simulink model "RealWorld"  (R2024b)
settings: Solver=VariableStepAuto  StartTime=0.0  StopTime=10.0  RelTol=1e-3
undefined symbols (not defined in the file or in its folder): env, flag, IC, orb, sat, sens
libraries: matrix_library x8, vrlib x1
(part 1 of 2)
settings Model: Creator=filippocamaleonte  LastModifiedBy=eleon

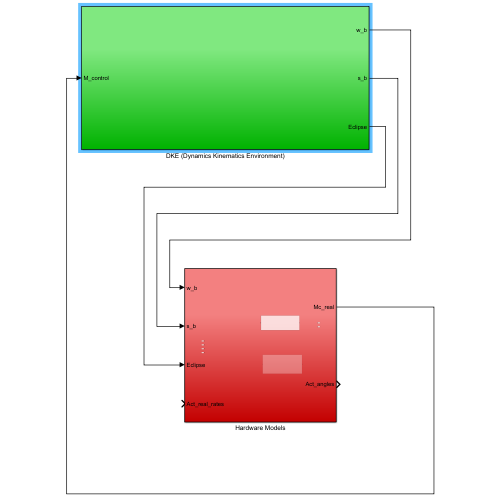
[thumbnail: Simulink's stored preview of the top-level diagram]
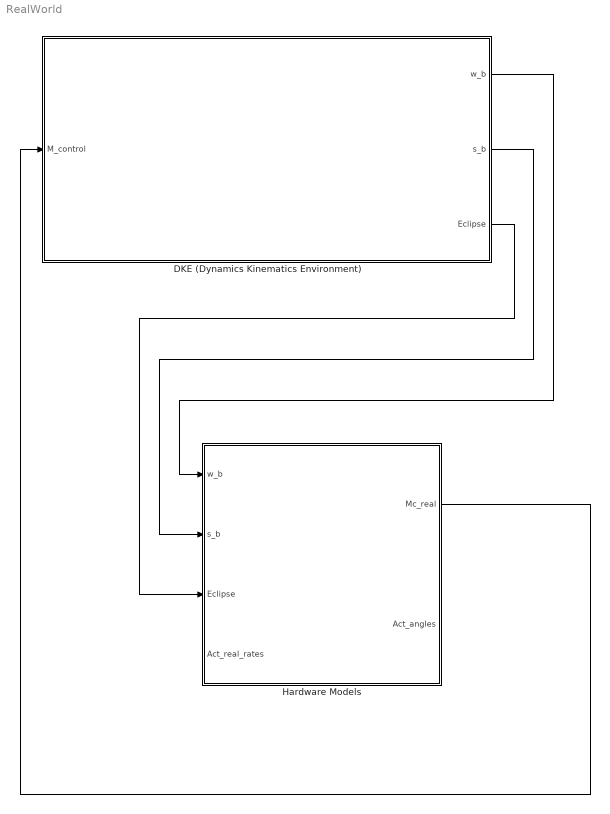
== system RealWorld ==
  DKE (Dynamics Kinematics Environment) : Subsystem
  Hardware Models : Subsystem
  wires:
  DKE (Dynamics Kinematics Environment)/2(s_b) -> Hardware Models/2(s_b)
  DKE (Dynamics Kinematics Environment)/3(Eclipse) -> Hardware Models/3(Eclipse)
  DKE (Dynamics Kinematics Environment)/1(w_b) -> Hardware Models/1(w_b)
  Hardware Models/1(Mc_real) -> DKE (Dynamics Kinematics Environment)/1(M_control)

== system RealWorld/DKE (Dynamics Kinematics Environment) ==
  M_control : Inport
  Dynamics : Subsystem
  Environment : Subsystem
  Kinematics : Subsystem
  Sum : Sum  Inputs=|++
  w_b : Outport
  s_b : Outport  Port=2
  Eclipse : Outport  Port=3
  wires:
  M_control/1 -> Sum/1
  Dynamics/1(w_b) -> [w_b], Kinematics/1(w_b)
  Sum/1 -> Dynamics/1(M_ext)
  Environment/3(Disturbance_torque) -> Sum/2
  [w_b] -> w_b/1
  Environment/1(Eclipse) -> Eclipse/1
  Kinematics/3(r_n) -> Environment/3(r_n)
  Kinematics/1(A_bn) -> Environment/1(A_bn)
  Kinematics/2(A_bl) -> Environment/2(A_bl)

== system RealWorld/Hardware Models ==
  w_b : Inport
  s_b : Inport  Port=2
  Eclipse : Inport  Port=3
  Act_real_rates : Inport  Port=4
  Actuators : Subsystem
  Sensors : Subsystem  Commented=on
  Mc_real : Outport
  Act_angles : Outport  Port=2

== system RealWorld/DKE (Dynamics Kinematics Environment)/Dynamics ==
  note: Here we need both Newton and Euler Law
  M_ext : Inport
  Euler Integrator : Subsystem
  w_b : Outport
  wires:
  M_ext/1 -> Euler Integrator/1(M_ext)
  Euler Integrator/1(w_b) -> w_b/1

== system RealWorld/DKE (Dynamics Kinematics Environment)/Environment ==
  note: Enviroment Models (Celestial Objects, Shadow, Magnetic Field, atmosphere, albedo)
  A_bn : Inport
  A_bl : Inport  Port=2
  r_n : Inport  Port=3
  Conical Shadow Model : Subsystem
  MatrixMultiply : Product  Multiplication=Matrix(*)
  Perturbations : Subsystem
  Sun Direction Circular Orbit : Subsystem
  Eclipse : Outport
  s_n : Outport  Port=2
  Disturbance_torque : Outport  Port=3
  wires:
  Sun Direction Circular Orbit/1(S_n) -> [S_n], s_n/1, Conical Shadow Model/1(S_n)
  Conical Shadow Model/1(eclipseFlag) -> Eclipse/1
  Perturbations/1(Disturbance_torque) -> Disturbance_torque/1
  r_n/1 -> Perturbations/2(r_n), Conical Shadow Model/2(r_n)
  A_bn/1 -> MatrixMultiply/1
  [S_n] -> MatrixMultiply/2
  MatrixMultiply/1 -> Perturbations/1(S_b)  "S_b"
  A_bl/1 -> Perturbations/3(A_bl)

== system RealWorld/DKE (Dynamics Kinematics Environment)/Kinematics ==
  note: B/N calculation
      | Keplerian calculations
      | L/N calculation
      | B/L calculation
  w_b : Inport
  Attitude Error : Subsystem
  Constant1 : Constant  Value=orb.i
  EulerKinematicsdelay : Subsystem
  Kepler Integrator1 : Subsystem
  LVLH Evolution wtr of Earth : Subsystem
  SpaceCraft position wrt ECI : Subsystem
  A_bn : Outport
  A_bl : Outport  Port=2
  r_n : Outport  Port=3
  wires:
  w_b/1 -> EulerKinematicsdelay/1(w_b)
  Attitude Error/1(A_bl) -> A_bl/1
  EulerKinematicsdelay/1(A_bn) -> A_bn/1, Attitude Error/1(A_bn)
  LVLH Evolution wtr of Earth/1(A_ln) -> Attitude Error/2(A_ln)
  Constant1/1 -> LVLH Evolution wtr of Earth/2(i)
  Kepler Integrator1/1(th) -> SpaceCraft position wrt ECI/1(th), LVLH Evolution wtr of Earth/1(th)
  SpaceCraft position wrt ECI/1(r_n) -> r_n/1

== system RealWorld/Hardware Models/Actuators ==
  In1 : Inport
  Out1 : Outport
  wires:
  In1/1 -> Out1/1

== system RealWorld/Hardware Models/Sensors ==
  note: Sun Sensors Array
  In1 : Inport
  Gyroscope : Subsystem
  Sun Sensor (S1) : Subsystem
  Sun Sensor (S2) : Subsystem
  Sun Sensor (S3) : Subsystem
  Sun Sensor (S4) : Subsystem
  Out1 : Outport

== system RealWorld/DKE (Dynamics Kinematics Environment)/Dynamics/Euler Integrator ==
  M_ext : Inport
  Constant : Constant  Value=sat.I
  Constant1 : Constant  Value=sat.w0  VectorParams1D=off
  Constant2 : Constant  Value=sat.invI
  Cross Product : matrix_library/Cross Product
  Divide : Product  Inputs=**  Multiplication=Matrix(*)
  Integrator : Integrator  InitialConditionSource=external
  Product : Product  Multiplication=Matrix(*)
  Sum : Sum  Inputs=|++
  w_b : Outport
  wires:
  Product/1 -> Cross Product/1
  Divide/1 -> Integrator/1
  Constant/1 -> Product/1
  Constant2/1 -> Divide/1
  Integrator/1 -> Product/2, Cross Product/2, w_b/1
  Constant1/1 -> Integrator/2
  Cross Product/1 -> Sum/1
  Sum/1 -> Divide/2
  M_ext/1 -> Sum/2

== system RealWorld/DKE (Dynamics Kinematics Environment)/Environment/Conical Shadow Model ==
  note: Output Interface
  note: Input Interface
  note: Model is cylindrical shadow, formula was taken by Crassidis
  S_n : Inport
  r_n : Inport  Port=2
  Dot Product : DotProduct  OutDataTypeStr=Inherit: Inherit via internal rule
  Earth's Radius : Constant  Value=env.Earth.R
  Eclipse (1) : Subsystem  TreatAsAtomicUnit=on
  Gain : Gain  Gain=-1
  If : If  NumInputs=2  IfExpression=u1 < u2
  Merge : Merge
  Norm : Subsystem
  NotEclipse (0) : Subsystem  TreatAsAtomicUnit=on
  Sqrt : Sqrt
  Square : Math  Operator=square
  Square1 : Math  Operator=square
  Subtract : Sum  Inputs=+-
  eclipseFlag : Outport
  wires:
  r_n/1 -> Dot Product/2, Norm/1(Vector)  "r_n"
  S_n/1 -> Dot Product/1  "S_n"
  Norm/1(Norm) -> Square1/1  "norm_r"
  If/1 -> Eclipse (1)/Action
  If/2 -> NotEclipse (0)/Action
  Merge/1 -> eclipseFlag/1
  Eclipse (1)/1(One) -> Merge/1
  NotEclipse (0)/1(Zero) -> Merge/2
  Dot Product/1 -> If/1
  Gain/1 -> If/2
  Sqrt/1 -> Gain/1
  Subtract/1 -> Sqrt/1
  Square/1 -> Subtract/2
  Square1/1 -> Subtract/1
  Earth's Radius/1 -> Square/1  "earth_R"

== system RealWorld/DKE (Dynamics Kinematics Environment)/Environment/Perturbations ==
  note: Gravity Gradiente
      | Solar Pressure
      | Magnetic torquer
      | Air drag ??
  S_b : Inport
  r_n : Inport  Port=2
  A_bl : Inport  Port=3
  Gravity Gradient Torque : Subsystem
  Magnetic Field order 1 : Subsystem
  Solar Radiation Pressure Torque : Subsystem
  Sum : Sum  Inputs=++++
  Disturbance_torque : Outport
  wires:
  Sum/1 -> Disturbance_torque/1
  Solar Radiation Pressure Torque/1(T_srp) -> Sum/2
  S_b/1 -> Solar Radiation Pressure Torque/1(S_b)
  A_bl/1 -> Gravity Gradient Torque/1(A_bl)
  r_n/1 -> Gravity Gradient Torque/2(r_n)
  Gravity Gradient Torque/1(T_gg) -> Sum/1

== system RealWorld/DKE (Dynamics Kinematics Environment)/Environment/Sun Direction Circular Orbit ==
  note: Input Interface
  note: Output Interface
  Clock : Clock
  Cos : Trigonometry  Operator=cos
  Cos1 : Trigonometry  Operator=cos
  Earth's Inclination : Constant  Value=env.Earth.i
  Gain : Gain  Gain=env.Earth.n
  Matrix Concatenate : Concatenate  NumInputs=3  Mode=Multidimensional array
  Product : Product
  Product1 : Product
  Product2 : Product
  Sin : Trigonometry
  Sin1 : Trigonometry
  Sun's Radius : Constant  Value=env.Sun.R
  S_n : Outport
  wires:
  Clock/1 -> Gain/1
  Gain/1 -> Sin/1, Cos/1
  Product/1 -> S_n/1
  Sun's Radius/1 -> Product/2
  Matrix Concatenate/1 -> Product/1
  Earth's Inclination/1 -> Sin1/1, Cos1/1
  Cos1/1 -> [cos]
  Sin1/1 -> [sin]
  Cos/1 -> Matrix Concatenate/1
  Product1/1 -> Matrix Concatenate/2
  Product2/1 -> Matrix Concatenate/3
  [sin] -> Product2/2
  [cos] -> Product1/1
  Sin/1 -> Product1/2, Product2/1

== system RealWorld/DKE (Dynamics Kinematics Environment)/Kinematics/Attitude Error ==
  A_bn : Inport
  A_ln : Inport  Port=2
  Matrix Multiply : Product  Multiplication=Matrix(*)
  Transpose : Math  Operator=transpose
  A_bl : Outport
  wires:
  Transpose/1 -> Matrix Multiply/2
  A_ln/1 -> Transpose/1
  Matrix Multiply/1 -> A_bl/1
  A_bn/1 -> Matrix Multiply/1

== system RealWorld/DKE (Dynamics Kinematics Environment)/Kinematics/EulerKinematicsdelay ==
  note: Logic
  note: The flag is set to -1 when 313 is used and to 1 when 312 is used
  w_b : Inport
  312 Propagator : Subsystem
  312To313 : Subsystem
  313 Propagator : Subsystem
  313To312 : Subsystem
  A312 : Subsystem
  A313 : Subsystem
  Abs : Abs  SaturateOnIntegerOverflow=off
  Cos : Trigonometry  Operator=cos
  IC : InitialCondition  Value=IC.angles
  IC1 : InitialCondition  Value=IC.angles
  IC3 : InitialCondition
  Relay : Relay  OnSwitchValue=0.75  OffSwitchValue=0.35  OffOutputValue=-1
  Selector1 : Selector  InputPortWidth=3  IndexOptions=Index vector (dialog)  Indices=[2]  OutputSizes=1
  Switch : Switch  Criteria=u2 > Threshold  SaturateOnIntegerOverflow=off  InputSameDT=off
  Switch1 : Switch  Criteria=u2 > Threshold  SaturateOnIntegerOverflow=off  InputSameDT=off
  To Workspace : ToWorkspace  VariableName=flag1  SampleTime=-1
  To Workspace1 : ToWorkspace  VariableName=eu312  SampleTime=-1
  To Workspace2 : ToWorkspace  VariableName=eu313  SampleTime=-1
  A_bn : Outport
  wires:
  Cos/1 -> Abs/1
  Selector1/1 -> Cos/1
  Abs/1 -> Relay/1
  A313/1(Out1) -> Switch/3
  w_b/1 -> 313 Propagator/2(w_b), 312 Propagator/2(w_b)  "w_b"
  313 Propagator/1(EA) -> [Euler313], A313/1(Euler Angles)  "EulerAngles313"
  A312/1(DCM) -> Switch/1
  Switch1/1 -> Selector1/1
  Switch/1 -> A_bn/1  "DCM"
  313To312/1(Out1) -> IC1/1
  312To313/1(Out1) -> IC/1
  IC1/1 -> 312 Propagator/1(IC)
  IC/1 -> 313 Propagator/3(IC)
  [EulerFlag] -> Switch/2, 312 Propagator/3(Reset), 313 Propagator/1(Reset)
  312 Propagator/1(EA) -> [Euler312], A312/1(Euler Angles)  "EulerAngles312"
  312 Propagator/2(Out1) -> 312To313/1(In1)
  313 Propagator/2(Out1) -> 313To312/1(In1)
  Relay/1 -> IC3/1
  [Euler312] -> To Workspace1/1, Switch1/1
  [Euler313] -> To Workspace2/1, Switch1/3
  [EulerFlag] -> Switch1/2
  IC3/1 -> To Workspace/1, [EulerFlag]

== system RealWorld/DKE (Dynamics Kinematics Environment)/Kinematics/Kepler Integrator1 ==
  Add : Sum  Inputs=+-
  Add1 : Sum
  Constant : Constant  Value=IC.theta
  Constant1 : Constant  Value=3/2
  Constant2 : Constant
  Constant3 : Constant  Value=2
  Constant4 : Constant  Value=orb.e
  Constant5 : Constant  Value=2
  Constant6 : Constant
  Cosh : Trigonometry  Operator=cos
  Divide : Product  Inputs=*/
  Gain : Gain  Gain=orb.n
  Gain1 : Gain  Gain=orb.e
  Integrator : Integrator  InitialConditionSource=external  WrapState=on  WrappedStateUpperValue=2*pi  WrappedStateLowerValue=0
  Power : Math  Operator=pow
  Power1 : Math  Operator=pow
  Power2 : Math  Operator=pow
  th : Outport
  wires:
  Constant/1 -> Integrator/2
  Integrator/1 -> Cosh/1, th/1
  Divide/1 -> Integrator/1
  Power/1 -> Divide/2
  Constant1/1 -> Power/2
  Constant2/1 -> Add/1
  Add/1 -> Power/1
  Power1/1 -> Add/2
  Constant3/1 -> Power1/2
  Constant4/1 -> Power1/1
  Gain/1 -> Divide/1
  Power2/1 -> Gain/1
  Constant5/1 -> Power2/2
  Add1/1 -> Power2/1
  Constant6/1 -> Add1/1
  Gain1/1 -> Add1/2
  Cosh/1 -> Gain1/1

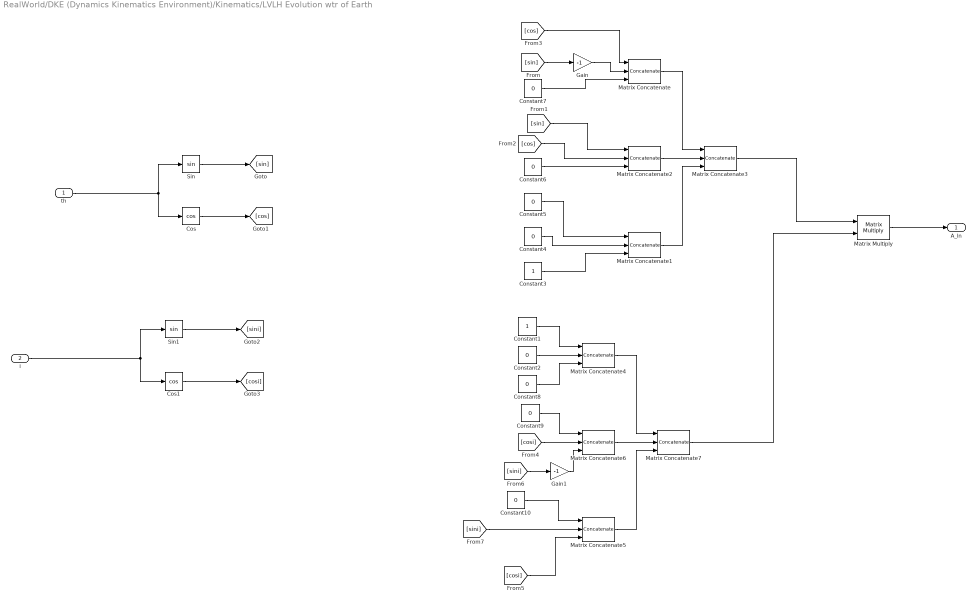
== system RealWorld/DKE (Dynamics Kinematics Environment)/Kinematics/LVLH Evolution wtr of Earth ==
  th : Inport
  i : Inport  Port=2
  Constant1 : Constant
  Constant{2,4..10} (8 alike) : Constant  Value=0
  Constant3 : Constant
  Cos : Trigonometry  Operator=cos
  Cos1 : Trigonometry  Operator=cos
  Gain : Gain  Gain=-1
  Gain1 : Gain  Gain=-1
  Matrix Concatenate{,1..2,4..6} (6 alike) : Concatenate  NumInputs=3  Mode=Multidimensional array
  Matrix Concatenate3 : Concatenate  NumInputs=3  Mode=Multidimensional array  ConcatenateDimension=2
  Matrix Concatenate7 : Concatenate  NumInputs=3  Mode=Multidimensional array  ConcatenateDimension=2
  Matrix Multiply : Product  Multiplication=Matrix(*)
  Sin : Trigonometry
  Sin1 : Trigonometry
  A_ln : Outport
  wires:
  Cos/1 -> [cos]
  Matrix Concatenate1/1 -> Matrix Concatenate3/3
  th/1 -> Cos/1, Sin/1
  Matrix Concatenate/1 -> Matrix Concatenate3/1
  Constant5/1 -> Matrix Concatenate1/1
  Constant3/1 -> Matrix Concatenate1/3
  [cos] -> Matrix Concatenate/1
  Sin/1 -> [sin]
  Constant6/1 -> Matrix Concatenate2/3
  Constant7/1 -> Matrix Concatenate/3
  Constant4/1 -> Matrix Concatenate1/2
  Matrix Concatenate2/1 -> Matrix Concatenate3/2
  [cos] -> Matrix Concatenate2/2
  [sin] -> Matrix Concatenate2/1
  Gain/1 -> Matrix Concatenate/2
  [sin] -> Gain/1
  Cos1/1 -> [cosi]
  Sin1/1 -> [sini]
  i/1 -> Cos1/1, Sin1/1
  Matrix Multiply/1 -> A_ln/1
  Matrix Concatenate3/1 -> Matrix Multiply/1
  Matrix Concatenate7/1 -> Matrix Multiply/2
  Matrix Concatenate6/1 -> Matrix Concatenate7/2
  Matrix Concatenate5/1 -> Matrix Concatenate7/3
  Matrix Concatenate4/1 -> Matrix Concatenate7/1
  Constant1/1 -> Matrix Concatenate4/1
  Constant2/1 -> Matrix Concatenate4/2
  Constant8/1 -> Matrix Concatenate4/3
  Constant9/1 -> Matrix Concatenate6/1
  Constant10/1 -> Matrix Concatenate5/1
  [cosi] -> Matrix Concatenate5/3
  [cosi] -> Matrix Concatenate6/2
  [sini] -> Matrix Concatenate5/2
  [sini] -> Gain1/1
  Gain1/1 -> Matrix Concatenate6/3

== system RealWorld/DKE (Dynamics Kinematics Environment)/Kinematics/SpaceCraft position wrt ECI ==
  th : Inport
  Add : Sum
  Add1 : Sum  Inputs=+-
  Constant : Constant  Value=orb.i
  Constant1 : Constant  Value=orb.i
  Constant2 : Constant
  Constant3 : Constant
  Constant4 : Constant  Value=2
  Constant5 : Constant  Value=orb.e
  Cos : Trigonometry  Operator=cos
  Cos1 : Trigonometry  Operator=cos
  Cos2 : Trigonometry  Operator=cos
  Divide : Product  Inputs=*/
  Gain : Gain  Gain=orb.e
  Gain1 : Gain  Gain=orb.a
  Matrix Concatenate : Concatenate  NumInputs=3  Mode=Multidimensional array
  Power : Math  Operator=pow
  Product : Product
  Product1 : Product
  Product2 : Product
  Sin : Trigonometry
  Sin1 : Trigonometry
  r_n : Outport
  wires:
  Constant/1 -> Sin/1
  Cos1/1 -> Matrix Concatenate/1
  th/1 -> Sin1/1, Cos2/1, Cos1/1
  Product1/1 -> Matrix Concatenate/2
  Product/1 -> Matrix Concatenate/3
  Sin1/1 -> Product1/2, Product/1
  Sin/1 -> Product/2
  Constant1/1 -> Cos/1
  Cos/1 -> Product1/1
  Product2/1 -> r_n/1
  Matrix Concatenate/1 -> Product2/1
  Divide/1 -> Product2/2
  Constant2/1 -> Add/1
  Add/1 -> Divide/2
  Cos2/1 -> Gain/1
  Gain/1 -> Add/2
  Constant3/1 -> Add1/1
  Power/1 -> Add1/2
  Constant4/1 -> Power/2
  Constant5/1 -> Power/1
  Add1/1 -> Gain1/1
  Gain1/1 -> Divide/1

== system RealWorld/Hardware Models/Sensors/Gyroscope ==
  note: Sensor Model
  note: Noise Model
  note: Input Interface
  note: G sensing Model
  note: Sources:
      | - Crassidis
      | - Giacomo Langfelder Course
      | - Colagrossi's book
      | - Safran STIM210 Datasheet
      |
      | To Do:
      | Add Temperature model and more precise dealy model
  note: We assume that the Sensor is Oriented in the same axis as the body
  note: Output Interface
  w_b : Inport
  a_b : Inport  Port=2
  Add : Sum  Inputs=++++
  Add1 : Sum
  Constant : Constant  Value=flag.realsensors
  Constant1 : Constant  Value=sens.gyro.scaleFactor
  Constant2 : Constant  Value=sens.gyro.orth
  Constant3 : Constant  Value=sens.gyro.missalign
  Constant4 : Constant  Value=sens.gyro.bias
  Constant5 : Constant  Value=sens.gyro.gsensing
  Discrete Transfer Fcn : DiscreteTransferFcn  Numerator=1  Denominator=[1 0.8]
  MatrixMultiply{,1..3} (4 alike) : Product  Multiplication=Matrix(*)
  Quantizer : Quantizer  QuantizationInterval=sens.gyro.ADC.quanta
  Random Number : RandomNumber  Variance=sens.gyro.biasInstability  SampleTime=1/sens.gyro.freq
  Random Number1 : RandomNumber  Variance=sens.gyro.arw  SampleTime=1/sens.gyro.freq
  Saturation : Saturate  UpperLimit=sens.gyro.saturation  LowerLimit=-sens.gyro.saturation
  Scope : Scope  NumInputPorts=2
  Scope1 : Scope
  Scope2 : Scope  NumInputPorts=2
  Switch : Switch  Criteria=u2 > Threshold  SaturateOnIntegerOverflow=off  InputSameDT=off
  Zero-Order Hold : ZeroOrderHold  SampleTime=1/sens.gyro.freq
  w_meas_b : Outport
  wires:
  Switch/1 -> w_meas_b/1
  Constant/1 -> Switch/2
  [w_meas_b] -> Switch/1
  [w_b] -> Switch/3
  w_b/1 -> [w_b]
  Quantizer/1 -> [w_meas_b]
  Zero-Order Hold/1 -> Quantizer/1
  Saturation/1 -> Zero-Order Hold/1
  MatrixMultiply/1 -> MatrixMultiply1/1
  MatrixMultiply1/1 -> MatrixMultiply2/1
  Constant1/1 -> MatrixMultiply/1
  Constant2/1 -> MatrixMultiply/2
  Constant3/1 -> MatrixMultiply1/2
  [w_b] -> MatrixMultiply2/2
  MatrixMultiply2/1 -> Add/1
  Add/1 -> Scope/1, Saturation/1
  Constant4/1 -> Add/2
  Add1/1 -> Scope1/1, [noise]
  [noise] -> Add/3
  MatrixMultiply3/1 -> Add/4
  a_b/1 -> [a_b]
  [a_b] -> MatrixMultiply3/2
  Constant5/1 -> MatrixMultiply3/1
  Discrete Transfer Fcn/1 -> Scope2/1, Add1/2
  Random Number/1 -> Discrete Transfer Fcn/1
  Random Number1/1 -> Scope2/2, Add1/1
  [w_b] -> Scope/2

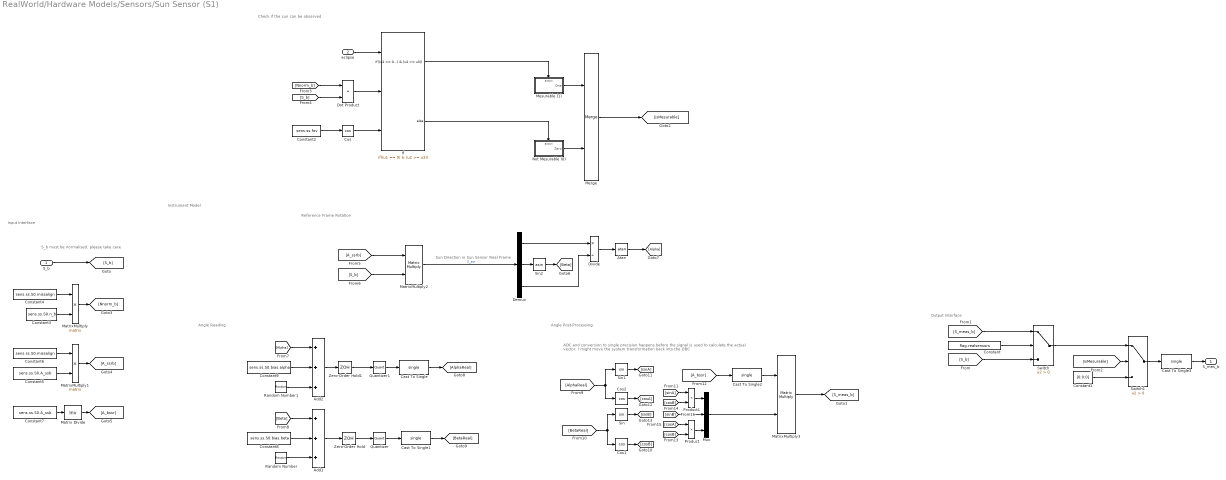
== system RealWorld/Hardware Models/Sensors/Sun Sensor (S1) ==
  note: Instrument Model
  note: Angle Reading
  note: Reference Frame Rotation
  note: ADC and conversion to single precision happens before the signal is used to calculate the actual vector. I might move the system transformation back into the OBC
  note: Sun Direction in Sun Sensor Real Frame
  note: S_b must be normalised, please take care
  note: Input Interface
  note: Output Interface
  note: Check if the sun can be observed
  note: Angle Post-Processing
  S_b : Inport
  eclipse : Inport  Port=2
  Add1 : Sum  Inputs=+++
  Add2 : Sum  Inputs=+++
  Atan : Trigonometry  Operator=atan
  Cast To Single{,1..3} (4 alike) : DataTypeConversion  OutDataTypeStr=single  SaturateOnIntegerOverflow=off  RndMeth=Floor
  Constant : Constant  Value=flag.realsensors
  Constant1 : Constant  Value=[0;0;0]
  Constant2 : Constant  Value=sens.ss.fov
  Constant3 : Constant  Value=sens.ss.S0.n_b
  Constant4 : Constant  Value=sens.ss.S0.missalign
  Constant5 : Constant  Value=sens.ss.S0.A_ssb
  Constant6 : Constant  Value=sens.ss.S0.missalign
  Constant7 : Constant  Value=sens.ss.S0.A_ssb
  Constant8 : Constant  Value=sens.ss.S0.bias.beta
  Constant9 : Constant  Value=sens.ss.S0.bias.alpha
  Cos : Trigonometry  Operator=cos
  Cos1 : Trigonometry  Operator=cos
  Cos2 : Trigonometry  Operator=cos
  Demux : Demux  Outputs=3
  Divide : Product  Inputs=*/
  Dot Product : DotProduct  OutDataTypeStr=Inherit: Inherit via internal rule
  If : If  NumInputs=3  IfExpression=(u1 == 0) & (u2 >= u3)
  Matrix Divide : Product  Inputs=/  Multiplication=Matrix(*)
  MatrixMultiply{,1..3} (4 alike) : Product  Multiplication=Matrix(*)
  Merge : Merge
  Mesurable (1) : Subsystem  TreatAsAtomicUnit=on
  Mux : Mux  Inputs=3
  Not Mesurable (0) : Subsystem  TreatAsAtomicUnit=on
  Product : Product
  Product1 : Product
  Quantizer : Quantizer  QuantizationInterval=sens.ss.ADC.quanta
  Quantizer1 : Quantizer  QuantizationInterval=sens.ss.ADC.quanta
  Random Number : RandomNumber  Variance=(sens.ss.precision/1.4)^2  Seed=sens.ss.S0.seed.beta  SampleTime=sens.ss.freq
  Random Number1 : RandomNumber  Variance=(sens.ss.precision/1.4)^2  Seed=sens.ss.S0.seed.beta  SampleTime=sens.ss.freq
  Sin : Trigonometry
  Sin1 : Trigonometry
  Sin2 : Trigonometry  Operator=asin
  Switch : Switch  Criteria=u2 > Threshold  SaturateOnIntegerOverflow=off  InputSameDT=off
  Switch1 : Switch  Criteria=u2 > Threshold  SaturateOnIntegerOverflow=off  InputSameDT=off
  Zero-Order Hold : ZeroOrderHold  SampleTime=sens.ss.freq
  Zero-Order Hold1 : ZeroOrderHold  SampleTime=sens.ss.freq
  S_mes_b : Outport
  wires:
  Constant/1 -> Switch/2
  S_b/1 -> [S_b]
  [S_b] -> Switch/3
  [S_meas_b] -> Switch/1
  eclipse/1 -> If/1
  If/1 -> Mesurable (1)/Action
  If/2 -> Not Mesurable (0)/Action
  Not Mesurable (0)/1(Zero) -> Merge/2
  Mesurable (1)/1(One) -> Merge/1
  Cos/1 -> If/3
  Constant2/1 -> Cos/1
  Dot Product/1 -> If/2
  Merge/1 -> [isMesurable]
  [isMesurable] -> Switch1/2
  [Nnorm_b] -> Dot Product/1
  [S_b] -> Dot Product/2
  Switch1/1 -> Cast To Single3/1
  Constant4/1 -> MatrixMultiply/1
  MatrixMultiply/1 -> [Nnorm_b]
  Constant3/1 -> MatrixMultiply/2
  Constant1/1 -> Switch1/3
  Switch/1 -> Switch1/1
  Constant6/1 -> MatrixMultiply1/1
  Constant5/1 -> MatrixMultiply1/2
  MatrixMultiply1/1 -> [A_ssrb]
  Constant7/1 -> Matrix Divide/1
  Matrix Divide/1 -> [A_bssr]
  [A_ssrb] -> MatrixMultiply2/1
  [S_b] -> MatrixMultiply2/2
  MatrixMultiply2/1 -> Demux/1  "S_ssr"
  Demux/1 -> Divide/1
  Demux/3 -> Divide/2
  Sin2/1 -> [Beta]
  Divide/1 -> Atan/1
  Add2/1 -> Zero-Order Hold1/1
  Add1/1 -> Zero-Order Hold/1
  Quantizer1/1 -> Cast To Single/1
  Zero-Order Hold1/1 -> Quantizer1/1
  Quantizer/1 -> Cast To Single1/1
  Zero-Order Hold/1 -> Quantizer/1
  [Alpha] -> Add2/1
  [Beta] -> Add1/1
  Constant8/1 -> Add1/2
  Constant9/1 -> Add2/2
  Cast To Single/1 -> [AlphaReal]
  Cast To Single1/1 -> [BetaReal]
  Random Number/1 -> Add1/3
  Random Number1/1 -> Add2/3
  Cast To Single3/1 -> S_mes_b/1
  MatrixMultiply3/1 -> [S_meas_b]
  Mux/1 -> MatrixMultiply3/2
  Cast To Single2/1 -> MatrixMultiply3/1
  [A_bssr] -> Cast To Single2/1
  [BetaReal] -> Cos1/1, Sin/1
  Atan/1 -> [Alpha]
  [AlphaReal] -> Cos2/1, Sin1/1
  Product/1 -> Mux/3
  Product1/1 -> Mux/1
  Demux/2 -> Sin2/1
  Sin1/1 -> [sinA]
  Cos2/1 -> [cosA]
  [sinA] -> Product1/1
  Cos1/1 -> [cosB]
  [cosB] -> Product/2
  [cosB] -> Product1/2
  [cosA] -> Product/1
  Sin/1 -> [sinB]
  [sinB] -> Mux/2

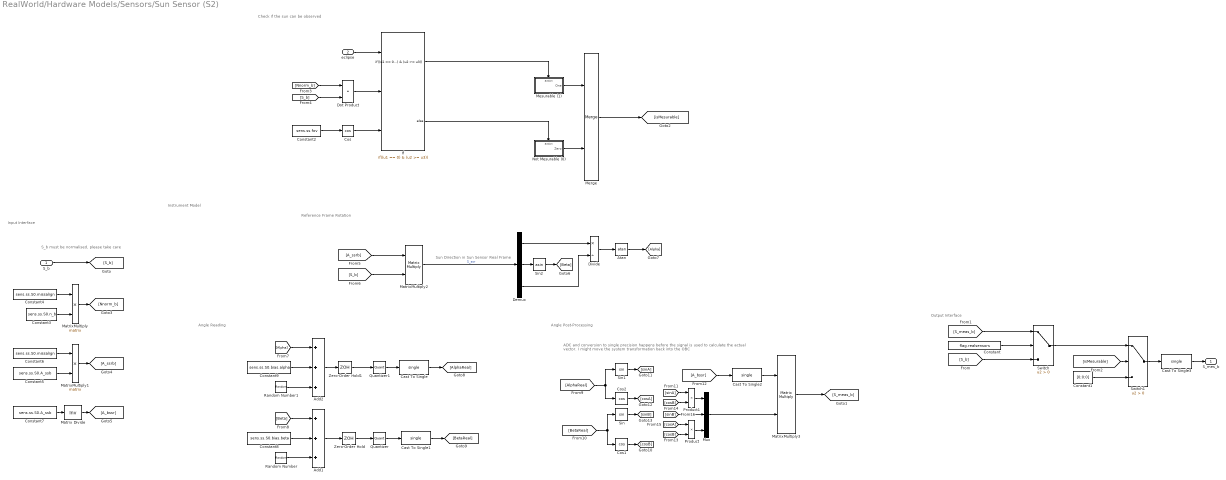
== system RealWorld/Hardware Models/Sensors/Sun Sensor (S2) ==
  note: Instrument Model
  note: Angle Reading
  note: Reference Frame Rotation
  note: ADC and conversion to single precision happens before the signal is used to calculate the actual vector. I might move the system transformation back into the OBC
  note: Sun Direction in Sun Sensor Real Frame
  note: S_b must be normalised, please take care
  note: Input Interface
  note: Output Interface
  note: Check if the sun can be observed
  note: Angle Post-Processing
  S_b : Inport
  eclipse : Inport  Port=2
  Add1 : Sum  Inputs=+++
  Add2 : Sum  Inputs=+++
  Atan : Trigonometry  Operator=atan
  Cast To Single{,1..3} (4 alike) : DataTypeConversion  OutDataTypeStr=single  SaturateOnIntegerOverflow=off  RndMeth=Floor
  Constant : Constant  Value=flag.realsensors
  Constant1 : Constant  Value=[0;0;0]
  Constant2 : Constant  Value=sens.ss.fov
  Constant3 : Constant  Value=sens.ss.S0.n_b
  Constant4 : Constant  Value=sens.ss.S0.missalign
  Constant5 : Constant  Value=sens.ss.S0.A_ssb
  Constant6 : Constant  Value=sens.ss.S0.missalign
  Constant7 : Constant  Value=sens.ss.S0.A_ssb
  Constant8 : Constant  Value=sens.ss.S0.bias.beta
  Constant9 : Constant  Value=sens.ss.S0.bias.alpha
  Cos : Trigonometry  Operator=cos
  Cos1 : Trigonometry  Operator=cos
  Cos2 : Trigonometry  Operator=cos
  Demux : Demux  Outputs=3
  Divide : Product  Inputs=*/
  Dot Product : DotProduct  OutDataTypeStr=Inherit: Inherit via internal rule
  If : If  NumInputs=3  IfExpression=(u1 == 0) & (u2 >= u3)
  Matrix Divide : Product  Inputs=/  Multiplication=Matrix(*)
  MatrixMultiply{,1..3} (4 alike) : Product  Multiplication=Matrix(*)
  Merge : Merge
  Mesurable (1) : Subsystem  TreatAsAtomicUnit=on
  Mux : Mux  Inputs=3
  Not Mesurable (0) : Subsystem  TreatAsAtomicUnit=on
  Product : Product
  Product1 : Product
  Quantizer : Quantizer  QuantizationInterval=sens.ss.ADC.quanta
  Quantizer1 : Quantizer  QuantizationInterval=sens.ss.ADC.quanta
  Random Number : RandomNumber  Variance=(sens.ss.precision/1.4)^2  Seed=sens.ss.S0.seed.beta  SampleTime=sens.ss.freq
  Random Number1 : RandomNumber  Variance=(sens.ss.precision/1.4)^2  Seed=sens.ss.S0.seed.beta  SampleTime=sens.ss.freq
  Sin : Trigonometry
  Sin1 : Trigonometry
  Sin2 : Trigonometry  Operator=asin
  Switch : Switch  Criteria=u2 > Threshold  SaturateOnIntegerOverflow=off  InputSameDT=off
  Switch1 : Switch  Criteria=u2 > Threshold  SaturateOnIntegerOverflow=off  InputSameDT=off
  Zero-Order Hold : ZeroOrderHold  SampleTime=sens.ss.freq
  Zero-Order Hold1 : ZeroOrderHold  SampleTime=sens.ss.freq
  S_mes_b : Outport
  wires:
  Constant/1 -> Switch/2
  S_b/1 -> [S_b]
  [S_b] -> Switch/3
  [S_meas_b] -> Switch/1
  eclipse/1 -> If/1
  If/1 -> Mesurable (1)/Action
  If/2 -> Not Mesurable (0)/Action
  Not Mesurable (0)/1(Zero) -> Merge/2
  Mesurable (1)/1(One) -> Merge/1
  Cos/1 -> If/3
  Constant2/1 -> Cos/1
  Dot Product/1 -> If/2
  Merge/1 -> [isMesurable]
  [isMesurable] -> Switch1/2
  [Nnorm_b] -> Dot Product/1
  [S_b] -> Dot Product/2
  Switch1/1 -> Cast To Single3/1
  Constant4/1 -> MatrixMultiply/1
  MatrixMultiply/1 -> [Nnorm_b]
  Constant3/1 -> MatrixMultiply/2
  Constant1/1 -> Switch1/3
  Switch/1 -> Switch1/1
  Constant6/1 -> MatrixMultiply1/1
  Constant5/1 -> MatrixMultiply1/2
  MatrixMultiply1/1 -> [A_ssrb]
  Constant7/1 -> Matrix Divide/1
  Matrix Divide/1 -> [A_bssr]
  [A_ssrb] -> MatrixMultiply2/1
  [S_b] -> MatrixMultiply2/2
  MatrixMultiply2/1 -> Demux/1  "S_ssr"
  Demux/1 -> Divide/1
  Demux/3 -> Divide/2
  Sin2/1 -> [Beta]
  Divide/1 -> Atan/1
  Add2/1 -> Zero-Order Hold1/1
  Add1/1 -> Zero-Order Hold/1
  Quantizer1/1 -> Cast To Single/1
  Zero-Order Hold1/1 -> Quantizer1/1
  Quantizer/1 -> Cast To Single1/1
  Zero-Order Hold/1 -> Quantizer/1
  [Alpha] -> Add2/1
  [Beta] -> Add1/1
  Constant8/1 -> Add1/2
  Constant9/1 -> Add2/2
  Cast To Single/1 -> [AlphaReal]
  Cast To Single1/1 -> [BetaReal]
  Random Number/1 -> Add1/3
  Random Number1/1 -> Add2/3
  Cast To Single3/1 -> S_mes_b/1
  MatrixMultiply3/1 -> [S_meas_b]
  Mux/1 -> MatrixMultiply3/2
  Cast To Single2/1 -> MatrixMultiply3/1
  [A_bssr] -> Cast To Single2/1
  [BetaReal] -> Cos1/1, Sin/1
  Atan/1 -> [Alpha]
  [AlphaReal] -> Cos2/1, Sin1/1
  Product/1 -> Mux/3
  Product1/1 -> Mux/1
  Demux/2 -> Sin2/1
  Sin1/1 -> [sinA]
  Cos2/1 -> [cosA]
  [sinA] -> Product1/1
  Cos1/1 -> [cosB]
  [cosB] -> Product/2
  [cosB] -> Product1/2
  [cosA] -> Product/1
  Sin/1 -> [sinB]
  [sinB] -> Mux/2

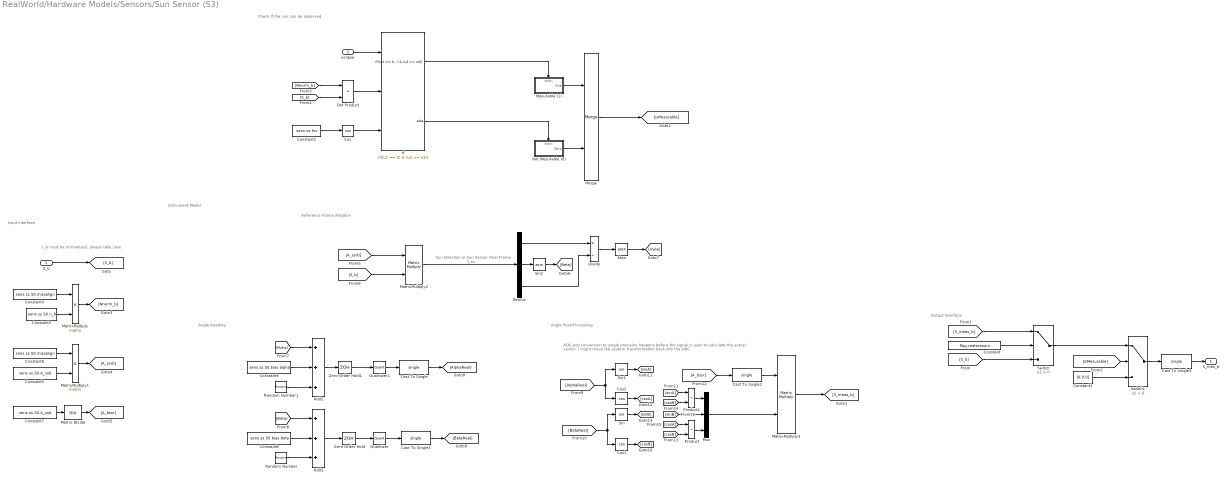
== system RealWorld/Hardware Models/Sensors/Sun Sensor (S3) ==
  note: Instrument Model
  note: Angle Reading
  note: Reference Frame Rotation
  note: ADC and conversion to single precision happens before the signal is used to calculate the actual vector. I might move the system transformation back into the OBC
  note: Sun Direction in Sun Sensor Real Frame
  note: S_b must be normalised, please take care
  note: Input Interface
  note: Output Interface
  note: Check if the sun can be observed
  note: Angle Post-Processing
  S_b : Inport
  eclipse : Inport  Port=2
  Add1 : Sum  Inputs=+++
  Add2 : Sum  Inputs=+++
  Atan : Trigonometry  Operator=atan
  Cast To Single{,1..3} (4 alike) : DataTypeConversion  OutDataTypeStr=single  SaturateOnIntegerOverflow=off  RndMeth=Floor
  Constant : Constant  Value=flag.realsensors
  Constant1 : Constant  Value=[0;0;0]
  Constant2 : Constant  Value=sens.ss.fov
  Constant3 : Constant  Value=sens.ss.S0.n_b
  Constant4 : Constant  Value=sens.ss.S0.missalign
  Constant5 : Constant  Value=sens.ss.S0.A_ssb
  Constant6 : Constant  Value=sens.ss.S0.missalign
  Constant7 : Constant  Value=sens.ss.S0.A_ssb
  Constant8 : Constant  Value=sens.ss.S0.bias.beta
  Constant9 : Constant  Value=sens.ss.S0.bias.alpha
  Cos : Trigonometry  Operator=cos
  Cos1 : Trigonometry  Operator=cos
  Cos2 : Trigonometry  Operator=cos
  Demux : Demux  Outputs=3
  Divide : Product  Inputs=*/
  Dot Product : DotProduct  OutDataTypeStr=Inherit: Inherit via internal rule
  If : If  NumInputs=3  IfExpression=(u1 == 0) & (u2 >= u3)
  Matrix Divide : Product  Inputs=/  Multiplication=Matrix(*)
  MatrixMultiply{,1..3} (4 alike) : Product  Multiplication=Matrix(*)
  Merge : Merge
  Mesurable (1) : Subsystem  TreatAsAtomicUnit=on
  Mux : Mux  Inputs=3
  Not Mesurable (0) : Subsystem  TreatAsAtomicUnit=on
  Product : Product
  Product1 : Product
  Quantizer : Quantizer  QuantizationInterval=sens.ss.ADC.quanta
  Quantizer1 : Quantizer  QuantizationInterval=sens.ss.ADC.quanta
  Random Number : RandomNumber  Variance=(sens.ss.precision/1.4)^2  Seed=sens.ss.S0.seed.beta  SampleTime=sens.ss.freq
  Random Number1 : RandomNumber  Variance=(sens.ss.precision/1.4)^2  Seed=sens.ss.S0.seed.beta  SampleTime=sens.ss.freq
  Sin : Trigonometry
  Sin1 : Trigonometry
  Sin2 : Trigonometry  Operator=asin
  Switch : Switch  Criteria=u2 > Threshold  SaturateOnIntegerOverflow=off  InputSameDT=off
  Switch1 : Switch  Criteria=u2 > Threshold  SaturateOnIntegerOverflow=off  InputSameDT=off
  Zero-Order Hold : ZeroOrderHold  SampleTime=sens.ss.freq
  Zero-Order Hold1 : ZeroOrderHold  SampleTime=sens.ss.freq
  S_mes_b : Outport
  wires:
  Constant/1 -> Switch/2
  S_b/1 -> [S_b]
  [S_b] -> Switch/3
  [S_meas_b] -> Switch/1
  eclipse/1 -> If/1
  If/1 -> Mesurable (1)/Action
  If/2 -> Not Mesurable (0)/Action
  Not Mesurable (0)/1(Zero) -> Merge/2
  Mesurable (1)/1(One) -> Merge/1
  Cos/1 -> If/3
  Constant2/1 -> Cos/1
  Dot Product/1 -> If/2
  Merge/1 -> [isMesurable]
  [isMesurable] -> Switch1/2
  [Nnorm_b] -> Dot Product/1
  [S_b] -> Dot Product/2
  Switch1/1 -> Cast To Single3/1
  Constant4/1 -> MatrixMultiply/1
  MatrixMultiply/1 -> [Nnorm_b]
  Constant3/1 -> MatrixMultiply/2
  Constant1/1 -> Switch1/3
  Switch/1 -> Switch1/1
  Constant6/1 -> MatrixMultiply1/1
  Constant5/1 -> MatrixMultiply1/2
  MatrixMultiply1/1 -> [A_ssrb]
  Constant7/1 -> Matrix Divide/1
  Matrix Divide/1 -> [A_bssr]
  [A_ssrb] -> MatrixMultiply2/1
  [S_b] -> MatrixMultiply2/2
  MatrixMultiply2/1 -> Demux/1  "S_ssr"
  Demux/1 -> Divide/1
  Demux/3 -> Divide/2
  Sin2/1 -> [Beta]
  Divide/1 -> Atan/1
  Add2/1 -> Zero-Order Hold1/1
  Add1/1 -> Zero-Order Hold/1
  Quantizer1/1 -> Cast To Single/1
  Zero-Order Hold1/1 -> Quantizer1/1
  Quantizer/1 -> Cast To Single1/1
  Zero-Order Hold/1 -> Quantizer/1
  [Alpha] -> Add2/1
  [Beta] -> Add1/1
  Constant8/1 -> Add1/2
  Constant9/1 -> Add2/2
  Cast To Single/1 -> [AlphaReal]
  Cast To Single1/1 -> [BetaReal]
  Random Number/1 -> Add1/3
  Random Number1/1 -> Add2/3
  Cast To Single3/1 -> S_mes_b/1
  MatrixMultiply3/1 -> [S_meas_b]
  Mux/1 -> MatrixMultiply3/2
  Cast To Single2/1 -> MatrixMultiply3/1
  [A_bssr] -> Cast To Single2/1
  [BetaReal] -> Cos1/1, Sin/1
  Atan/1 -> [Alpha]
  [AlphaReal] -> Cos2/1, Sin1/1
  Product/1 -> Mux/3
  Product1/1 -> Mux/1
  Demux/2 -> Sin2/1
  Sin1/1 -> [sinA]
  Cos2/1 -> [cosA]
  [sinA] -> Product1/1
  Cos1/1 -> [cosB]
  [cosB] -> Product/2
  [cosB] -> Product1/2
  [cosA] -> Product/1
  Sin/1 -> [sinB]
  [sinB] -> Mux/2

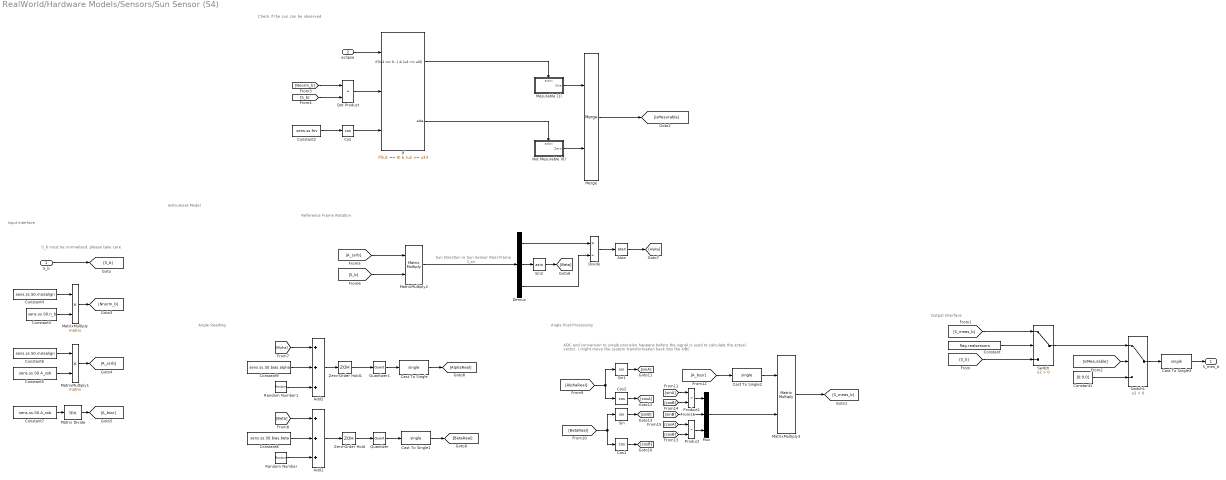
== system RealWorld/Hardware Models/Sensors/Sun Sensor (S4) ==
  note: Instrument Model
  note: Angle Reading
  note: Reference Frame Rotation
  note: ADC and conversion to single precision happens before the signal is used to calculate the actual vector. I might move the system transformation back into the OBC
  note: Sun Direction in Sun Sensor Real Frame
  note: S_b must be normalised, please take care
  note: Input Interface
  note: Output Interface
  note: Check if the sun can be observed
  note: Angle Post-Processing
  S_b : Inport
  eclipse : Inport  Port=2
  Add1 : Sum  Inputs=+++
  Add2 : Sum  Inputs=+++
  Atan : Trigonometry  Operator=atan
  Cast To Single{,1..3} (4 alike) : DataTypeConversion  OutDataTypeStr=single  SaturateOnIntegerOverflow=off  RndMeth=Floor
  Constant : Constant  Value=flag.realsensors
  Constant1 : Constant  Value=[0;0;0]
  Constant2 : Constant  Value=sens.ss.fov
  Constant3 : Constant  Value=sens.ss.S0.n_b
  Constant4 : Constant  Value=sens.ss.S0.missalign
  Constant5 : Constant  Value=sens.ss.S0.A_ssb
  Constant6 : Constant  Value=sens.ss.S0.missalign
  Constant7 : Constant  Value=sens.ss.S0.A_ssb
  Constant8 : Constant  Value=sens.ss.S0.bias.beta
  Constant9 : Constant  Value=sens.ss.S0.bias.alpha
  Cos : Trigonometry  Operator=cos
  Cos1 : Trigonometry  Operator=cos
  Cos2 : Trigonometry  Operator=cos
  Demux : Demux  Outputs=3
  Divide : Product  Inputs=*/
  Dot Product : DotProduct  OutDataTypeStr=Inherit: Inherit via internal rule
  If : If  NumInputs=3  IfExpression=(u1 == 0) & (u2 >= u3)
  Matrix Divide : Product  Inputs=/  Multiplication=Matrix(*)
  MatrixMultiply{,1..3} (4 alike) : Product  Multiplication=Matrix(*)
  Merge : Merge
  Mesurable (1) : Subsystem  TreatAsAtomicUnit=on
  Mux : Mux  Inputs=3
  Not Mesurable (0) : Subsystem  TreatAsAtomicUnit=on
  Product : Product
  Product1 : Product
  Quantizer : Quantizer  QuantizationInterval=sens.ss.ADC.quanta
  Quantizer1 : Quantizer  QuantizationInterval=sens.ss.ADC.quanta
  Random Number : RandomNumber  Variance=(sens.ss.precision/1.4)^2  Seed=sens.ss.S0.seed.beta  SampleTime=sens.ss.freq
  Random Number1 : RandomNumber  Variance=(sens.ss.precision/1.4)^2  Seed=sens.ss.S0.seed.beta  SampleTime=sens.ss.freq
  Sin : Trigonometry
  Sin1 : Trigonometry
  Sin2 : Trigonometry  Operator=asin
  Switch : Switch  Criteria=u2 > Threshold  SaturateOnIntegerOverflow=off  InputSameDT=off
  Switch1 : Switch  Criteria=u2 > Threshold  SaturateOnIntegerOverflow=off  InputSameDT=off
  Zero-Order Hold : ZeroOrderHold  SampleTime=sens.ss.freq
  Zero-Order Hold1 : ZeroOrderHold  SampleTime=sens.ss.freq
  S_mes_b : Outport
  wires:
  Constant/1 -> Switch/2
  S_b/1 -> [S_b]
  [S_b] -> Switch/3
  [S_meas_b] -> Switch/1
  eclipse/1 -> If/1
  If/1 -> Mesurable (1)/Action
  If/2 -> Not Mesurable (0)/Action
  Not Mesurable (0)/1(Zero) -> Merge/2
  Mesurable (1)/1(One) -> Merge/1
  Cos/1 -> If/3
  Constant2/1 -> Cos/1
  Dot Product/1 -> If/2
  Merge/1 -> [isMesurable]
  [isMesurable] -> Switch1/2
  [Nnorm_b] -> Dot Product/1
  [S_b] -> Dot Product/2
  Switch1/1 -> Cast To Single3/1
  Constant4/1 -> MatrixMultiply/1
  MatrixMultiply/1 -> [Nnorm_b]
  Constant3/1 -> MatrixMultiply/2
  Constant1/1 -> Switch1/3
  Switch/1 -> Switch1/1
  Constant6/1 -> MatrixMultiply1/1
  Constant5/1 -> MatrixMultiply1/2
  MatrixMultiply1/1 -> [A_ssrb]
  Constant7/1 -> Matrix Divide/1
  Matrix Divide/1 -> [A_bssr]
  [A_ssrb] -> MatrixMultiply2/1
  [S_b] -> MatrixMultiply2/2
  MatrixMultiply2/1 -> Demux/1  "S_ssr"
  Demux/1 -> Divide/1
  Demux/3 -> Divide/2
  Sin2/1 -> [Beta]
  Divide/1 -> Atan/1
  Add2/1 -> Zero-Order Hold1/1
  Add1/1 -> Zero-Order Hold/1
  Quantizer1/1 -> Cast To Single/1
  Zero-Order Hold1/1 -> Quantizer1/1
  Quantizer/1 -> Cast To Single1/1
  Zero-Order Hold/1 -> Quantizer/1
  [Alpha] -> Add2/1
  [Beta] -> Add1/1
  Constant8/1 -> Add1/2
  Constant9/1 -> Add2/2
  Cast To Single/1 -> [AlphaReal]
  Cast To Single1/1 -> [BetaReal]
  Random Number/1 -> Add1/3
  Random Number1/1 -> Add2/3
  Cast To Single3/1 -> S_mes_b/1
  MatrixMultiply3/1 -> [S_meas_b]
  Mux/1 -> MatrixMultiply3/2
  Cast To Single2/1 -> MatrixMultiply3/1
  [A_bssr] -> Cast To Single2/1
  [BetaReal] -> Cos1/1, Sin/1
  Atan/1 -> [Alpha]
  [AlphaReal] -> Cos2/1, Sin1/1
  Product/1 -> Mux/3
  Product1/1 -> Mux/1
  Demux/2 -> Sin2/1
  Sin1/1 -> [sinA]
  Cos2/1 -> [cosA]
  [sinA] -> Product1/1
  Cos1/1 -> [cosB]
  [cosB] -> Product/2
  [cosB] -> Product1/2
  [cosA] -> Product/1
  Sin/1 -> [sinB]
  [sinB] -> Mux/2

== system RealWorld/DKE (Dynamics Kinematics Environment)/Environment/Conical Shadow Model/Eclipse (1) ==
  Action Port : ActionPort
  Constant : Constant
  One : Outport
  wires:
  Constant/1 -> One/1

== system RealWorld/DKE (Dynamics Kinematics Environment)/Environment/Conical Shadow Model/Norm ==
  Vector : Inport
  Add : Sum  Inputs=+++
  Demux : Demux  Outputs=3
  Sqrt : Sqrt
  Square : Math  Operator=square
  Square1 : Math  Operator=square
  Square2 : Math  Operator=square
  Norm : Outport
  wires:
  Square/1 -> Add/1
  Add/1 -> Sqrt/1
  Demux/3 -> Square1/1
  Square2/1 -> Add/2
  Square1/1 -> Add/3
  Demux/1 -> Square/1
  Demux/2 -> Square2/1
  Vector/1 -> Demux/1
  Sqrt/1 -> Norm/1

== system RealWorld/DKE (Dynamics Kinematics Environment)/Environment/Conical Shadow Model/NotEclipse (0) ==
  Action Port : ActionPort
  Constant : Constant  Value=0
  Zero : Outport
  wires:
  Constant/1 -> Zero/1

== system RealWorld/DKE (Dynamics Kinematics Environment)/Environment/Perturbations/Gravity Gradient Torque ==
  A_bl : Inport
  r_n : Inport  Port=2
  Constant : Constant  Value=[0; 0; 0]
  Constant1 : Constant  Value=flag.gg
  Constant3 : Constant  Value=3
  Constant5 : Constant  Value=env.Earth.mass
  Constant6 : Constant  Value=env.G
  Constant7 : Constant  Value=[1; 0; 0]
  Constant8 : Constant  Value=sat.I
  Cross Product1 : matrix_library/Cross Product
  Divide1 : Product  Inputs=**/
  Gain : Gain  Gain=3
  Power : Math  Operator=pow
  Product1 : Product
  Product2 : Product  Multiplication=Matrix(*)
  Product3 : Product  Multiplication=Matrix(*)
  Switch : Switch  Criteria=u2 > Threshold  SaturateOnIntegerOverflow=off  InputSameDT=off
  T_gg : Outport
  wires:
  A_bl/1 -> Product2/1
  Product3/1 -> Cross Product1/2
  Product2/1 -> [c]
  Constant8/1 -> Product3/1
  Product1/1 -> Cross Product1/1
  [c] -> Product1/1
  [c] -> Product3/2
  Constant6/1 -> Divide1/1
  Constant5/1 -> Divide1/2
  r_n/1 -> Power/1
  Constant7/1 -> Product2/2
  Constant3/1 -> Power/2
  Power/1 -> Divide1/3
  Divide1/1 -> Gain/1
  Gain/1 -> Product1/2
  Constant/1 -> Switch/3
  Switch/1 -> T_gg/1
  Cross Product1/1 -> Switch/1
  Constant1/1 -> Switch/2

== system RealWorld/DKE (Dynamics Kinematics Environment)/Environment/Perturbations/Magnetic Field order 1 ==
  r_n : Inport
  Clock : Clock
  Constant : Constant  Value=env.mag.dgrf2020
  Constant1 : Constant  Value=env.Earth.R
  Constant2 : Constant  Value=3
  Constant3 : Constant  Value=env.Earth.magInclination
  Constant4 : Constant  Value=3
  Cos : Trigonometry  Operator=cos
  Cos1 : Trigonometry  Operator=cos
  Divide : Product  Inputs=***/
  Divide1 : Product  Inputs=*/
  Divide2 : Product  Inputs=*/
  Dot Product : DotProduct  OutDataTypeStr=Inherit: Inherit via internal rule
  Gain : Gain  Gain=3
  Gain1 : Gain  Gain=env.Earth.omega
  Mux : Mux  Inputs=3
  Norm : Subsystem
  Norm1 : Subsystem
  Norm2 : Subsystem
  Power : Math  Operator=pow
  Power1 : Math  Operator=pow
  Product : Product
  Product1 : Product
  Product2 : Product
  Sin : Trigonometry
  Sin1 : Trigonometry
  Sqrt : Sqrt
  Square : Math  Operator=square
  Subtract : Sum  Inputs=+-
  Sum of Elements : Sum  Inputs=+
  Out1 : Outport
  wires:
  Constant/1 -> Square/1
  Square/1 -> Sum of Elements/1
  Sum of Elements/1 -> Sqrt/1
  Constant1/1 -> Power/1
  Constant2/1 -> Power/2
  Sqrt/1 -> Divide/2
  Power/1 -> Divide/3
  Constant4/1 -> Power1/2
  Power1/1 -> Divide/4
  Norm/1(Norm) -> Power1/1  "norm_r"
  r_n/1 -> Norm2/1(Vector), Divide2/1, [rr]
  [rr] -> Norm/1(Vector)
  [rr_hat] -> Dot Product/2
  Subtract/1 -> Divide/1
  [mm] -> Subtract/2
  Dot Product/1 -> Product/2
  Product/1 -> Gain/1
  Gain/1 -> Subtract/1
  [rr_hat] -> Product/1
  [mm] -> Dot Product/1
  Mux/1 -> Norm1/1(Vector), Divide1/1
  Cos/1 -> Mux/3
  Constant3/1 -> Sin/1, Cos/1
  Clock/1 -> Gain1/1
  Sin/1 -> Product2/2, Product1/2
  Product1/1 -> Mux/2
  Product2/1 -> Mux/1
  Cos1/1 -> Product2/1
  Gain1/1 -> Cos1/1, Sin1/1
  Sin1/1 -> Product1/1
  Divide/1 -> Out1/1
  Norm1/1(Norm) -> Divide1/2  "norm_r"
  Divide1/1 -> [mm]
  Norm2/1(Norm) -> Divide2/2  "norm_r"
  Divide2/1 -> [rr_hat]

== system RealWorld/DKE (Dynamics Kinematics Environment)/Environment/Perturbations/Solar Radiation Pressure Torque ==
  S_b : Inport
  Constant : Constant  Value=flag.srp
  Constant1 : Constant  Value=[0; 0; 0]
  Constant3 : Constant  Value=ones(6,1)-sat.rho_s
  Constant4 : Constant  Value=sat.rho_s
  Constant5 : Constant  Value=sat.rho_d
  Gain1 : Gain  Gain=-env.dis.P
  Gain2 : Gain  Gain=2
  Gain3 : Gain  Gain=2/3
  Matrix Concatenate : Concatenate  NumInputs=3  Mode=Multidimensional array
  Matrix Concatenate2 : Concatenate  NumInputs=3  Mode=Multidimensional array
  MatrixMultiply : Product  Multiplication=Matrix(*)
  Normalize Vector : vrlib/Utilities/Normalize Vector  maxzero=0
  Product{,1,3..4} (4 alike) : Product
  Product2 : Product  Multiplication=Matrix(*)
  Saturation : Saturate  UpperLimit=1  LowerLimit=0
  Sum1 : Sum  Inputs=+|+
  Sum2 : Sum  Inputs=+|+
  Switch : Switch  Criteria=u2 > Threshold  SaturateOnIntegerOverflow=off  InputSameDT=off
  Transpose : Math  Operator=transpose
  Transpose2 : Math  Operator=transpose
  Transpose3 : Math  Operator=transpose
  cross product r x F : Subsystem
  surface : Constant  Value=sat.A
  unit vector matrix : Constant  Value=sat.n_b
  T_srp : Outport
  wires:
  Product3/1 -> Transpose3/1
  Saturation/1 -> Product4/2, Product1/1
  Gain3/1 -> Sum1/2
  surface/1 -> Gain1/1
  unit vector matrix/1 -> MatrixMultiply/2, Product/2
  Constant4/1 -> Gain2/1
  Constant3/1 -> Product2/1
  Sum2/1 -> Product3/2
  [S_b] -> Product2/2
  Constant5/1 -> Gain3/1
  Product4/1 -> Sum1/1
  MatrixMultiply/1 -> Saturation/1
  Gain2/1 -> Product4/1
  Product2/1 -> Transpose/1
  S_b/1 -> Normalize Vector/1
  Normalize Vector/1 -> Transpose2/1
  Transpose2/1 -> MatrixMultiply/1, [S_b]
  Product/1 -> Sum2/2
  Transpose/1 -> Sum2/1
  Transpose3/1 -> cross product r x F/1(F_srp)
  Gain1/1 -> Product1/2
  Sum1/1 -> Matrix Concatenate/3, Matrix Concatenate/1, Matrix Concatenate/2
  Matrix Concatenate/1 -> Product/1
  Product1/1 -> Matrix Concatenate2/3, Matrix Concatenate2/2, Matrix Concatenate2/1
  Matrix Concatenate2/1 -> Product3/1
  cross product r x F/1(Out1) -> Switch/1
  Constant/1 -> Switch/2
  Switch/1 -> T_srp/1
  Constant1/1 -> Switch/3

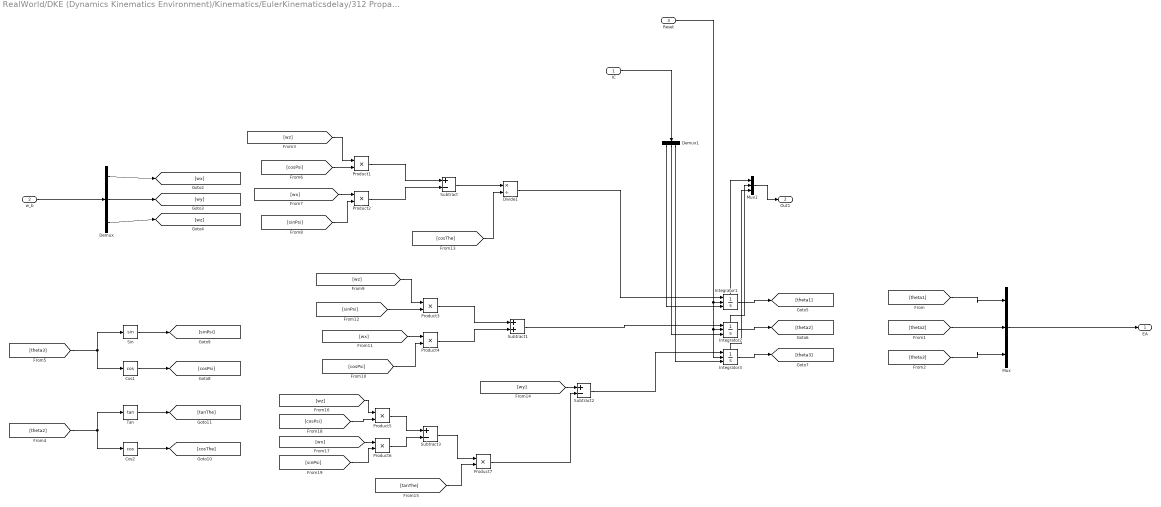
== system RealWorld/DKE (Dynamics Kinematics Environment)/Kinematics/EulerKinematicsdelay/312 Propagator ==
  IC : Inport
  w_b : Inport  Port=2
  Reset : Inport  Port=3
  Cos1 : Trigonometry  Operator=cos
  Cos2 : Trigonometry  Operator=cos
  Demux : Demux  Outputs=3
  Demux1 : Demux  Outputs=3
  Divide1 : Product  Inputs=*/
  Integrator1 : Integrator  ExternalReset=either  InitialConditionSource=external  WrapState=on  WrappedStateUpperValue=2*pi  WrappedStateLowerValue=0  ShowStatePort=on
  Integrator2 : Integrator  ExternalReset=either  InitialConditionSource=external  WrapState=on  ShowStatePort=on
  Integrator3 : Integrator  ExternalReset=either  InitialConditionSource=external  WrapState=on  WrappedStateUpperValue=2*pi  WrappedStateLowerValue=0  ShowStatePort=on
  Mux : Mux  Inputs=3
  Mux1 : Mux  Inputs=3
  Product{1..7} (7 alike) : Product
  Sin : Trigonometry
  Subtract : Sum  Inputs=+-
  Subtract1 : Sum
  Subtract2 : Sum  Inputs=+-
  Subtract3 : Sum  Inputs=+-
  Tan : Trigonometry  Operator=tan
  EA : Outport
  Out1 : Outport  Port=2
  wires:
  Product6/1 -> Subtract3/2
  Product5/1 -> Subtract3/1
  Product4/1 -> Subtract1/2
  Integrator3/1 -> [theta3]
  [wz] -> Product5/1
  Mux/1 -> EA/1
  Product7/1 -> Subtract2/2
  Cos1/1 -> [cosPsi]
  [theta3] -> Sin/1, Cos1/1
  [cosPsi] -> Product1/2
  Demux/2 -> [wy]
  Tan/1 -> [tanThe]
  Product2/1 -> Subtract/2
  [wz] -> Product3/1
  [tanThe] -> Product7/2
  Cos2/1 -> [cosThe]
  [cosPsi] -> Product5/2
  Divide1/1 -> Integrator1/1
  Subtract1/1 -> Integrator2/1
  Demux/3 -> [wz]
  [theta1] -> Mux/1
  Subtract/1 -> Divide1/1
  Demux/1 -> [wx]
  Subtract2/1 -> Integrator3/1
  [theta2] -> Tan/1, Cos2/1
  [wy] -> Subtract2/1
  Integrator1/1 -> [theta1]
  Integrator2/1 -> [theta2]
  [wx] -> Product4/1
  [sinPsi] -> Product2/2
  w_b/1 -> Demux/1
  Subtract3/1 -> Product7/1
  Product3/1 -> Subtract1/1
  [theta2] -> Mux/2
  [sinPsi] -> Product3/2
  [theta3] -> Mux/3
  [sinPsi] -> Product6/2
  [wx] -> Product6/1
  [wx] -> Product2/1
  [cosPsi] -> Product4/2
  [wz] -> Product1/1
  Product1/1 -> Subtract/1
  [cosThe] -> Divide1/2
  Sin/1 -> [sinPsi]
  Demux1/1 -> Integrator1/3
  Demux1/2 -> Integrator2/3
  Demux1/3 -> Integrator3/3
  IC/1 -> Demux1/1
  Reset/1 -> Integrator2/2, Integrator3/2, Integrator1/2
  Integrator3/State -> Mux1/3
  Integrator2/State -> Mux1/2
  Integrator1/State -> Mux1/1
  Mux1/1 -> Out1/1

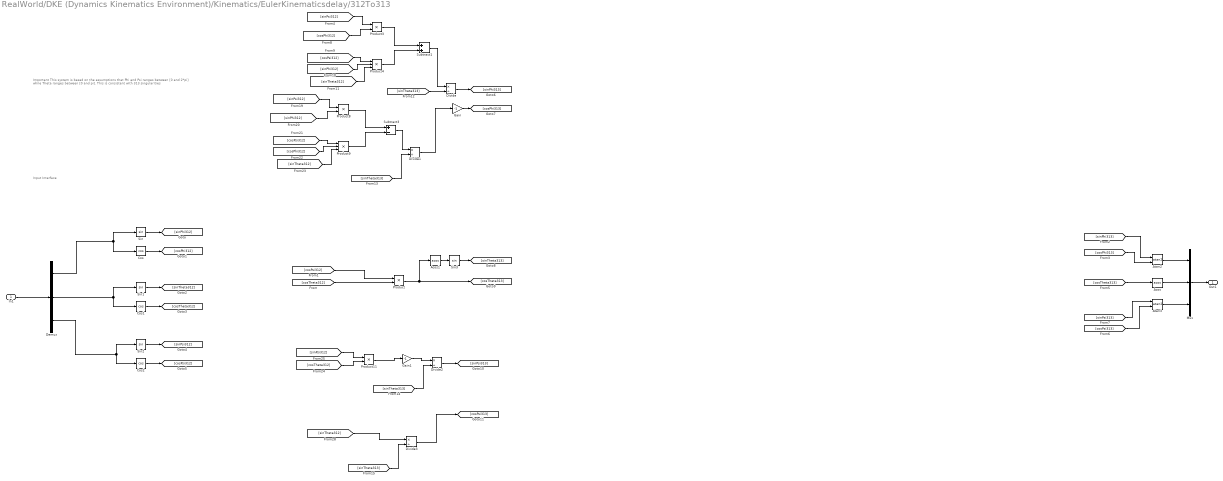
== system RealWorld/DKE (Dynamics Kinematics Environment)/Kinematics/EulerKinematicsdelay/312To313 ==
  note: Important
      |
      | This system is based on the assumptions that Phi and Psi ranges between [0 and 2*pi] while Theta ranges between [0 and pi]. This is consistent with 313 singularities
  note: Input Interface
  In1 : Inport
  Acos : Trigonometry  Operator=acos
  Acos1 : Trigonometry  Operator=acos
  Atan2 : Trigonometry  Operator=atan2
  Atan3 : Trigonometry  Operator=atan2
  Cos : Trigonometry  Operator=cos
  Cos1 : Trigonometry  Operator=cos
  Cos2 : Trigonometry  Operator=cos
  Demux : Demux  Outputs=3
  Divide{,1..3} (4 alike) : Product  Inputs=*/
  Gain : Gain  Gain=-1
  Gain1 : Gain  Gain=-1
  Mux : Mux  Inputs=3
  Product{,3,8,11} (4 alike) : Product
  Product4 : Product  Inputs=3
  Product9 : Product  Inputs=3
  Sin{,1..3} (4 alike) : Trigonometry
  Subtract1 : Sum
  Subtract3 : Sum  Inputs=+-
  Out1 : Outport
  wires:
  In1/1 -> Demux/1
  Mux/1 -> Out1/1
  Sin/1 -> [sinPhi312]
  Cos/1 -> [cosPhi312]
  Demux/1 -> Sin/1, Cos/1
  Sin1/1 -> [sinTheta312]
  Demux/2 -> Sin1/1, Cos1/1
  Cos1/1 -> [cosTheta312]
  Sin2/1 -> [sinPsi312]
  Cos2/1 -> [cosPsi312]
  Demux/3 -> Sin2/1, Cos2/1
  Product/1 -> Acos1/1, [cosTheta313]
  [cosTheta312] -> Product/2
  [cosPsi312] -> Product/1
  Atan2/1 -> Mux/1
  Acos/1 -> Mux/2
  Atan3/1 -> Mux/3
  [sinPhi313] -> Atan2/1
  [cosPhi313] -> Atan2/2
  [cosTheta313] -> Acos/1
  [cosPsi313] -> Atan3/2
  [sinPsi313] -> Atan3/1
  Sin3/1 -> [sinTheta313]
  Acos1/1 -> Sin3/1
  [cosPsi312] -> Product4/1
  [sinTheta312] -> Product4/3
  Product3/1 -> Subtract1/1
  [cosPhi312] -> Product3/2
  Product4/1 -> Subtract1/2
  [sinPsi312] -> Product3/1
  [sinPhi312] -> Product4/2
  Divide/1 -> [sinPhi313]
  [sinTheta313] -> Divide/2
  Subtract1/1 -> Divide/1
  Gain/1 -> [cosPhi313]
  Divide1/1 -> Gain/1
  [sinTheta313] -> Divide1/2
  [cosPsi312] -> Product9/1
  Product9/1 -> Subtract3/2
  Subtract3/1 -> Divide1/1
  [sinPsi312] -> Product8/1
  [cosPhi312] -> Product9/2
  [sinPhi312] -> Product8/2
  [sinTheta312] -> Product9/3
  Product8/1 -> Subtract3/1
  [sinTheta313] -> Divide2/2
  Divide2/1 -> [sinPsi313]
  [sinTheta313] -> Divide3/2
  Divide3/1 -> [cosPsi313]
  Product11/1 -> Gain1/1
  [sinPsi312] -> Product11/1
  [cosTheta312] -> Product11/2
  Gain1/1 -> Divide2/1
  [sinTheta312] -> Divide3/1

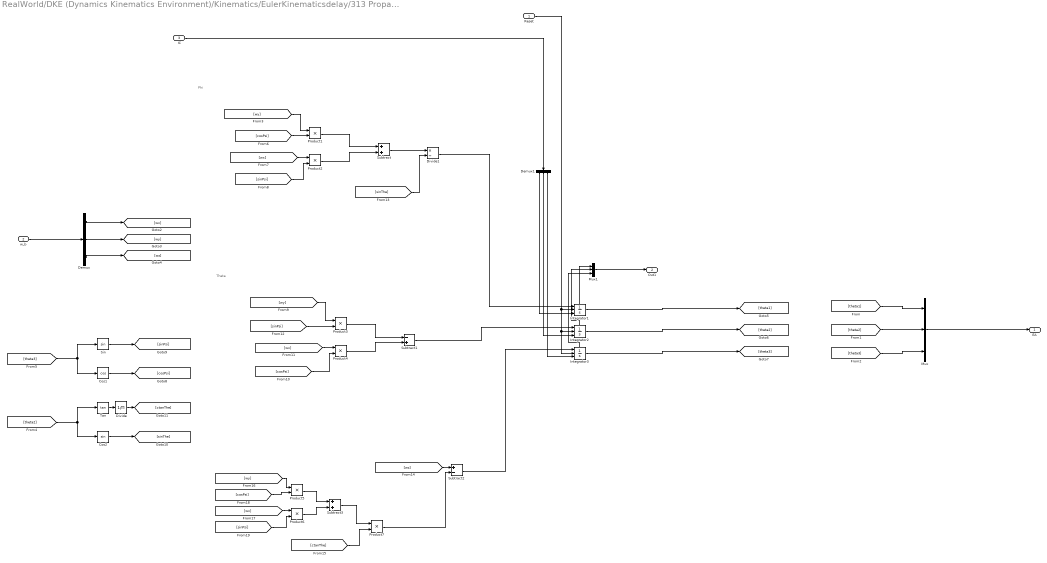
== system RealWorld/DKE (Dynamics Kinematics Environment)/Kinematics/EulerKinematicsdelay/313 Propagator ==
  note: Phi
  note: Theta
  Reset : Inport
  w_b : Inport  Port=2
  IC : Inport  Port=3
  Cos1 : Trigonometry  Operator=cos
  Cos2 : Trigonometry
  Demux : Demux  Outputs=3
  Demux1 : Demux  Outputs=3
  Divide : Product  Inputs=/
  Divide1 : Product  Inputs=*/
  Integrator1 : Integrator  ExternalReset=either  InitialConditionSource=external  WrapState=on  WrappedStateUpperValue=2*pi  WrappedStateLowerValue=0  ShowStatePort=on
  Integrator2 : Integrator  ExternalReset=either  InitialConditionSource=external  InitialCondition=pi/4  WrapState=on  ShowStatePort=on
  Integrator3 : Integrator  ExternalReset=either  InitialConditionSource=external  WrapState=on  WrappedStateUpperValue=2*pi  WrappedStateLowerValue=0  ShowStatePort=on
  Mux : Mux  Inputs=3
  Mux1 : Mux  Inputs=3
  Product{1..7} (7 alike) : Product
  Sin : Trigonometry
  Subtract : Sum
  Subtract1 : Sum  Inputs=-+
  Subtract2 : Sum  Inputs=+-
  Subtract3 : Sum
  Tan : Trigonometry  Operator=tan
  EA : Outport
  Out1 : Outport  Port=2
  wires:
  [sinThe] -> Divide1/2
  Sin/1 -> [sinPsi]
  [wx] -> Product2/1
  [theta3] -> Mux/3
  [theta2] -> Mux/2
  Product3/1 -> Subtract1/1
  w_b/1 -> Demux/1
  [sinPsi] -> Product3/2
  [sinPsi] -> Product6/2
  Subtract3/1 -> Product7/1
  Product1/1 -> Subtract/1
  [wx] -> Product6/1
  [wy] -> Product1/1
  [wz] -> Subtract2/1
  Subtract2/1 -> Integrator3/1
  [theta2] -> Tan/1, Cos2/1
  [cosPsi] -> Product4/2
  Demux/1 -> [wx]
  [sinPsi] -> Product2/2
  Integrator2/1 -> [theta2]
  [wx] -> Product4/1
  Tan/1 -> Divide/1
  [cosPsi] -> Product1/2
  Divide1/1 -> Integrator1/1
  Integrator1/1 -> [theta1]
  [ctanThe] -> Product7/2
  [cosPsi] -> Product5/2
  [wy] -> Product3/1
  Product2/1 -> Subtract/2
  Demux/2 -> [wy]
  Product5/1 -> Subtract3/1
  [wy] -> Product5/1
  Integrator3/1 -> [theta3]
  Product6/1 -> Subtract3/2
  Mux/1 -> EA/1
  Product4/1 -> Subtract1/2
  [theta3] -> Sin/1, Cos1/1
  Product7/1 -> Subtract2/2
  Cos2/1 -> [sinThe]
  Subtract1/1 -> Integrator2/1
  [theta1] -> Mux/1
  Subtract/1 -> Divide1/1
  Demux/3 -> [wz]
  Cos1/1 -> [cosPsi]
  Divide/1 -> [ctanThe]
  Demux1/3 -> Integrator3/3
  Demux1/2 -> Integrator2/3
  Demux1/1 -> Integrator1/3
  IC/1 -> Demux1/1
  Reset/1 -> Integrator1/2, Integrator2/2, Integrator3/2
  Integrator3/State -> Mux1/3
  Integrator2/State -> Mux1/2
  Mux1/1 -> Out1/1
  Integrator1/State -> Mux1/1
